simulink model "Project1Part1_"  (R2023b)
settings: Solver=ode1  StartTime=0.0  StopTime=25  FixedStep=0.1  RelTol=1e-3
values from neighbouring files (symbols this model uses):
  A = 1    [Project1Week2.m]    (also in ProjectWeek1.m; Project_1.m = 4)
  b = 1    [Project1Week2.m]    (also in ProjectWeek1.m; Project_1.m)
  F = 0    [Project1Final.m]
  isSin = 1    [Project1Final.m]
  w_0 = 1    [Project1Week2.m]    (also in ProjectWeek1.m; Project_1.m)
undefined symbols (not defined in the file or in its folder): J1
settings Model: Creator=Julian Tan  LastModifiedBy=hasch

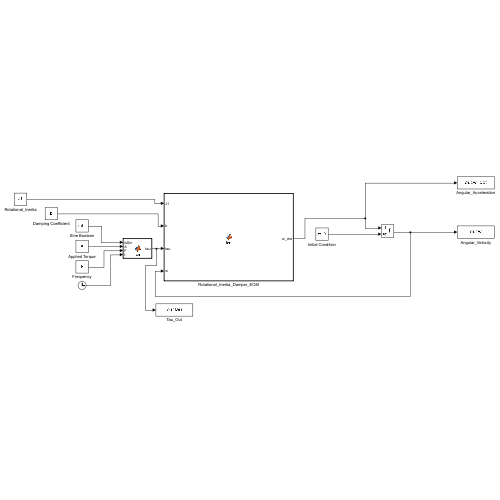
[thumbnail: Simulink's stored preview of the top-level diagram]
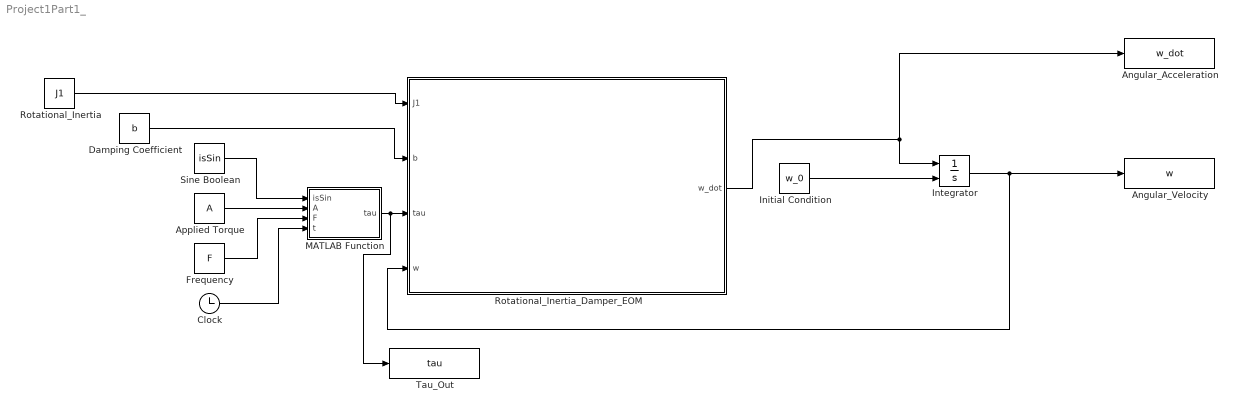
== system Project1Part1_ ==
  Angular_Acceleration : ToWorkspace  VariableName=w_dot  SaveFormat=Timeseries  SampleTime=-1
  Angular_Velocity : ToWorkspace  VariableName=w  SaveFormat=Timeseries  SampleTime=-1
  Applied Torque : Constant  Value=A
  Clock : Clock
  Damping Coefficient : Constant  Value=b
  Frequency : Constant  Value=F
  Initial Condition : Constant  Value=w_0
  Integrator : Integrator  InitialConditionSource=external  LimitOutput=on  UpperSaturationLimit=10
  MATLAB Function : MATLAB Function  TreatAsAtomicUnit=on
  Rotational_Inertia : Constant  Value=J1
  Rotational_Inertia_Damper_EOM : MATLAB Function  TreatAsAtomicUnit=on
  Sine Boolean : Constant  Value=isSin
  Tau_Out : ToWorkspace  VariableName=tau  SaveFormat=Timeseries  SampleTime=-1
  wires:
  Rotational_Inertia_Damper_EOM/1(w_dot) -> Angular_Acceleration/1, Integrator/1
  Applied Torque/1 -> MATLAB Function/2(A)
  Initial Condition/1 -> Integrator/2
  Damping Coefficient/1 -> Rotational_Inertia_Damper_EOM/2(b)
  Integrator/1 -> Angular_Velocity/1, Rotational_Inertia_Damper_EOM/4(w)
  Rotational_Inertia/1 -> Rotational_Inertia_Damper_EOM/1(J1)
  Clock/1 -> MATLAB Function/4(t)
  Frequency/1 -> MATLAB Function/3(F)
  MATLAB Function/1(tau) -> Tau_Out/1, Rotational_Inertia_Damper_EOM/3(tau)
  Sine Boolean/1 -> MATLAB Function/1(isSin)

== matlab function Project1Part1_/MATLAB Function ==
  data: isSin input; tau output; A input; F input; t input
function tau = fcn(isSin, A, F, t)

if isSin == 0
    tau = A;
else
    tau = A*sin(F*t);
end

== matlab function Project1Part1_/Rotational_Inertia_Damper_EOM ==
  data: J1 input; w_dot output; b input; tau input; w input
function w_dot = fcn(J1, b, tau, w)

tau_damped = b*w;
w_dot = (1/J1)*(tau - tau_damped);

end
